simulink model "Diagrama_motor"  (R2014a)
settings: Solver=ode15s  StartTime=0.0  StopTime=1  MaxStep=0.001  RelTol=1e-3
values from neighbouring files (symbols this model uses):
  b = 1.1    [TP1.m]
  J = 15    [TP1.m]
  K = 6.7628    [TP1.m]
  L = 2.886e-3    (= 0.002886)    [TP1.m]    (also in retrato3d.m = W\A*W)
  R = 50.296e-3    (= 0.050296)    [TP1.m]
settings Model: Creator=lraff  LastModifiedBy=lraff
settings DataIOCC: LimitDataPoints=off

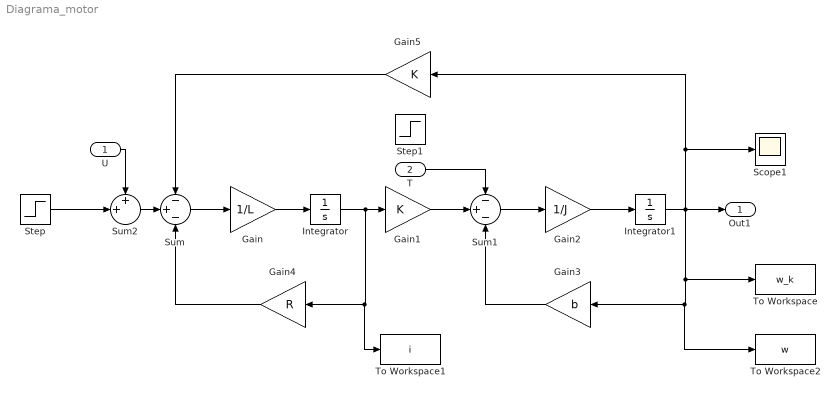
== system Diagrama_motor ==
  U : Inport
  T : Inport  Port=2
  Gain : Gain  Gain=1/L
  Gain1 : Gain  Gain=K
  Gain2 : Gain  Gain=1/J
  Gain3 : Gain  Gain=b
  Gain4 : Gain  Gain=R
  Gain5 : Gain  Gain=K
  Integrator : Integrator
  Integrator1 : Integrator
  Scope1 : Scope
  Step : Step  Time=0  After=440  SampleTime=0
  Step1 : Step  Time=0  After=5000  SampleTime=0
  Sum : Sum  Inputs=-+-
  Sum1 : Sum  Inputs=-+-
  Sum2 : Sum  Inputs=++|
  To Workspace : ToWorkspace  VariableName=w_k  SaveFormat=Timeseries  SampleTime=0.01
  To Workspace1 : ToWorkspace  VariableName=i  SaveFormat=Timeseries  SampleTime=-1
  To Workspace2 : ToWorkspace  VariableName=w  SaveFormat=Timeseries  SampleTime=-1
  Out1 : Outport
  wires:
  Sum/1 -> Gain/1
  Gain/1 -> Integrator/1
  Integrator/1 -> To Workspace1/1, Gain4/1, Gain1/1
  Gain1/1 -> Sum1/2
  Sum1/1 -> Gain2/1
  Gain2/1 -> Integrator1/1
  Integrator1/1 -> Out1/1, Scope1/1, Gain5/1, To Workspace/1, To Workspace2/1, Gain3/1
  Gain3/1 -> Sum1/3
  Gain4/1 -> Sum/3
  Gain5/1 -> Sum/1
  T/1 -> Sum1/1
  Step/1 -> Sum2/2
  U/1 -> Sum2/1
  Sum2/1 -> Sum/2
